simulink model "hardware5"  (R2021a)
settings: Solver=FixedStepAuto  StartTime=0.0  StopTime=1  FixedStep=0.001  RelTol=1e-3
undefined symbols (not defined in the file or in its folder): DiscIntNeverNeededParam
libraries: simulink x3
settings Model: Creator=acre  LastModifiedBy=acre
settings OptimizationCC: BlockReduction=off  OptimizeBlockIOStorage=off

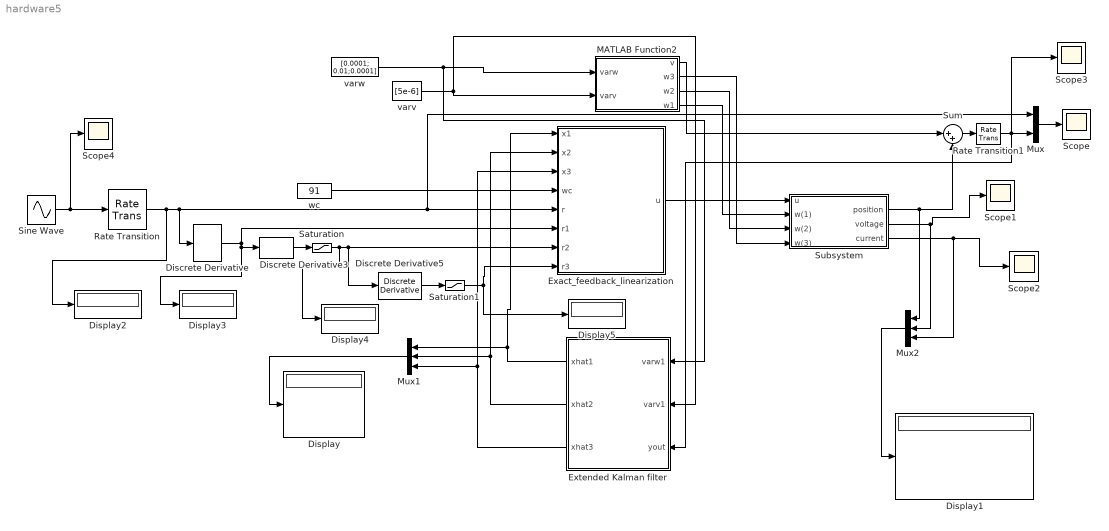
== system hardware5 ==
  Discrete Derivative : simulink/Discrete/Discrete Derivative  gainval=1.0  ICPrevScaledInput=0  OutMin=[]  OutMax=[]  OutDataType=fixdt(1, 16)  OutScaling=2^-10  DoSatur=off
  Discrete Derivative3 : simulink/Discrete/Discrete Derivative  gainval=1.0  ICPrevScaledInput=0  OutMin=[-1]  OutMax=[1]  OutDataType=fixdt(1, 16)  OutScaling=2^-10  DoSatur=on
      settings: LockScale=on
  Discrete Derivative5 : simulink/Discrete/Discrete Derivative  gainval=1.0  ICPrevScaledInput=0  OutMin=[]  OutMax=[]  OutDataType=fixdt(1, 16)  OutScaling=2^-10  DoSatur=off
  Display{,1..5} (6 alike) : Display
  Exact_feedback_linearization : Subsystem
  Extended Kalman filter : Subsystem
  MATLAB Function2 : MATLAB Function  TreatAsAtomicUnit=on
  Mux : Mux  Inputs=2
  Mux1 : Mux  Inputs=3
  Mux2 : Mux  Inputs=3
  Rate Transition : RateTransition
  Rate Transition1 : RateTransition
  Saturation : Saturate  UpperLimit=1  LowerLimit=-1
  Saturation1 : Saturate  UpperLimit=4  LowerLimit=-4
  Scope{,1..4} (5 alike) : Scope
  Sine Wave : Sin  Amplitude=0.1  Frequency=3  SampleTime=0
  Subsystem : Subsystem
  Sum : Sum  Inputs=|++
  varv : Constant  Value=[5e-6]  SampleTime=-1
  varw : Constant  Value=[0.0001; 0.01;0.0001]  SampleTime=-1
  wc : Constant  Value=91
  wires:
  Discrete Derivative3/1 -> Saturation/1
  Sine Wave/1 -> Scope4/1, Rate Transition/1
  Exact_feedback_linearization/1(u) -> Subsystem/1(u)
  Extended Kalman filter/3(xhat3) -> Mux1/3, Exact_feedback_linearization/3(x3)
  MATLAB Function2/2(w3) -> Subsystem/4(w(3))
  Mux1/1 -> Display/1
  Discrete Derivative5/1 -> Saturation1/1
  Rate Transition/1 -> Display2/1, Mux/1, Exact_feedback_linearization/5(r), Discrete Derivative/1
  Sum/1 -> Rate Transition1/1
  Mux/1 -> Scope/1
  Extended Kalman filter/1(xhat1) -> Exact_feedback_linearization/1(x1), Mux1/1
  MATLAB Function2/1(v) -> Sum/1
  varv/1 -> MATLAB Function2/2(varv), Extended Kalman filter/2(varv1)
  Saturation/1 -> Display4/1, Discrete Derivative5/1, Exact_feedback_linearization/7(r2)
  Rate Transition1/1 -> Extended Kalman filter/3(yout), Scope3/1, Mux/2
  Discrete Derivative/1 -> Display3/1, Discrete Derivative3/1, Exact_feedback_linearization/6(r1)
  wc/1 -> Exact_feedback_linearization/4(wc)
  MATLAB Function2/3(w2) -> Subsystem/3(w(2))
  Extended Kalman filter/2(xhat2) -> Mux1/2, Exact_feedback_linearization/2(x2)
  MATLAB Function2/4(w1) -> Subsystem/2(w(1))
  varw/1 -> Extended Kalman filter/1(varw1), MATLAB Function2/1(varw)
  Saturation1/1 -> Exact_feedback_linearization/8(r3), Display5/1
  Subsystem/1(position) -> Mux2/1, Sum/2
  Subsystem/2(voltage) -> Mux2/2, Scope1/1
  Subsystem/3(current) -> Mux2/3, Scope2/1
  Mux2/1 -> Display1/1

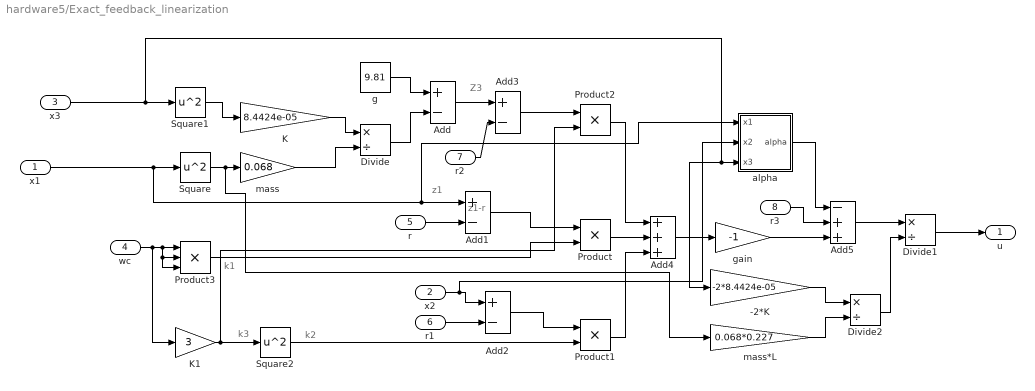
== system hardware5/Exact_feedback_linearization ==
  note: z1
  note: z1-r
  note: k3
  note: k2
  note: k1
  note: Z3
  x1 : Inport
  x2 : Inport  Port=2
  x3 : Inport  Port=3
  wc : Inport  Port=4
  r : Inport  Port=5
  r1 : Inport  Port=6
  r2 : Inport  Port=7
  r3 : Inport  Port=8
  -2*K : Gain  Gain=-2*8.4424e-05
  Add{,1..3} (4 alike) : Sum  Inputs=+-
  Add4 : Sum  Inputs=+++
  Add5 : Sum  Inputs=-++
  Divide : Product  Inputs=*/
  Divide1 : Product  Inputs=*/
  Divide2 : Product  Inputs=*/
  K : Gain  Gain=8.4424e-05
  K1 : Gain  Gain=3
  Product : Product
  Product1 : Product
  Product2 : Product
  Product3 : Product  Inputs=3
  Square : Math  Operator=square  SaturateOnIntegerOverflow=on
  Square1 : Math  Operator=square  SaturateOnIntegerOverflow=on
  Square2 : Math  Operator=square  SaturateOnIntegerOverflow=on
  alpha : Subsystem
  g : Constant  Value=9.81
  gain : Gain  Gain=-1
  mass : Gain  Gain=0.068
  mass*L : Gain  Gain=0.068*0.227
  u : Outport
  wires:
  g/1 -> Add/1
  Divide/1 -> Add/2
  Square1/1 -> K/1
  K/1 -> Divide/1
  mass/1 -> Divide/2
  wc/1 -> Product3/3, Product3/2, Product3/1, K1/1
  K1/1 -> Product2/2, Square2/1
  r/1 -> Add1/2
  Add1/1 -> Product/1
  Product3/1 -> Product/2
  r1/1 -> Add2/2
  x2/1 -> alpha/2(x2), Add2/1
  Add2/1 -> Product1/1
  Square2/1 -> Product1/2
  Add/1 -> Add3/1
  r2/1 -> Add3/2
  Add3/1 -> Product2/1
  Product2/1 -> Add4/1
  Product/1 -> Add4/2
  Product1/1 -> Add4/3
  Add4/1 -> gain/1
  gain/1 -> Add5/3
  r3/1 -> Add5/2
  Add5/1 -> Divide1/1
  Divide1/1 -> u/1
  Square/1 -> mass*L/1, mass/1
  -2*K/1 -> Divide2/1
  mass*L/1 -> Divide2/2
  Divide2/1 -> Divide1/2
  alpha/1(alpha) -> Add5/1
  x1/1 -> alpha/1(x1), Add1/1, Square/1
  x3/1 -> alpha/3(x3), -2*K/1, Square1/1

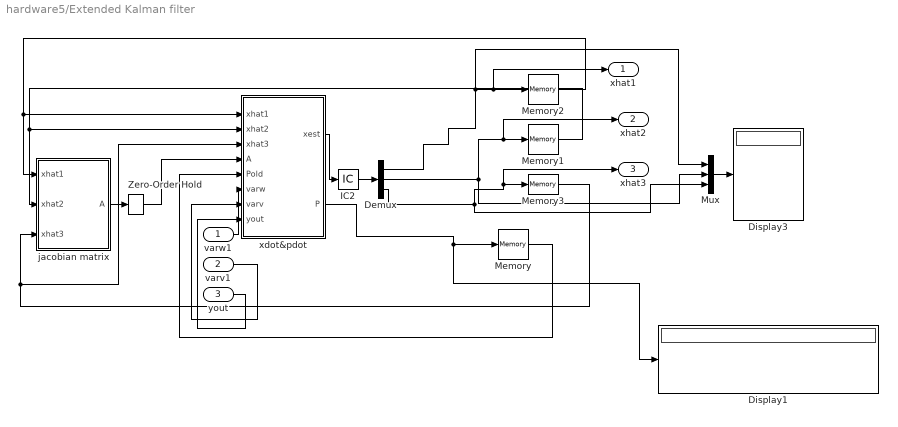
== system hardware5/Extended Kalman filter ==
  varw1 : Inport
  varv1 : Inport  Port=2
  yout : Inport  Port=3
  Demux : Demux  Outputs=3
  Display1 : Display
  Display3 : Display
  IC2 : InitialCondition  Value=[0.0095;0;0.84]
  Memory : Memory  InitialCondition=[0.00003 0 0;0 0.1 0;0 0 10]
  Memory1 : Memory  InitialCondition=0.0001
  Memory2 : Memory  InitialCondition=0.0095
  Memory3 : Memory  InitialCondition=0.84
  Mux : Mux  Inputs=3
  Zero-Order Hold : ZeroOrderHold  SampleTime=0.001
  jacobian matrix : MATLAB Function  TreatAsAtomicUnit=on
  xdot&pdot : MATLAB Function  TreatAsAtomicUnit=on
  xhat1 : Outport
  xhat2 : Outport  Port=2
  xhat3 : Outport  Port=3
  wires:
  varv1/1 -> xdot&pdot/7(varv)
  varw1/1 -> xdot&pdot/6(varw)
  Memory1/1 -> jacobian matrix/2(xhat2), xdot&pdot/2(xhat2)
  xdot&pdot/1(xest) -> IC2/1
  Memory2/1 -> jacobian matrix/1(xhat1), xdot&pdot/1(xhat1)
  Memory3/1 -> jacobian matrix/3(xhat3), xdot&pdot/3(xhat3)
  jacobian matrix/1(A) -> Zero-Order Hold/1
  Memory/1 -> xdot&pdot/5(Pold)
  yout/1 -> xdot&pdot/8(yout)
  Mux/1 -> Display3/1
  xdot&pdot/2(P) -> Display1/1, Memory/1
  Zero-Order Hold/1 -> xdot&pdot/4(A)
  Demux/1 -> Mux/1, xhat1/1, Memory2/1
  Demux/2 -> xhat2/1, Memory1/1, Mux/2
  Demux/3 -> Memory3/1, xhat3/1, Mux/3
  IC2/1 -> Demux/1

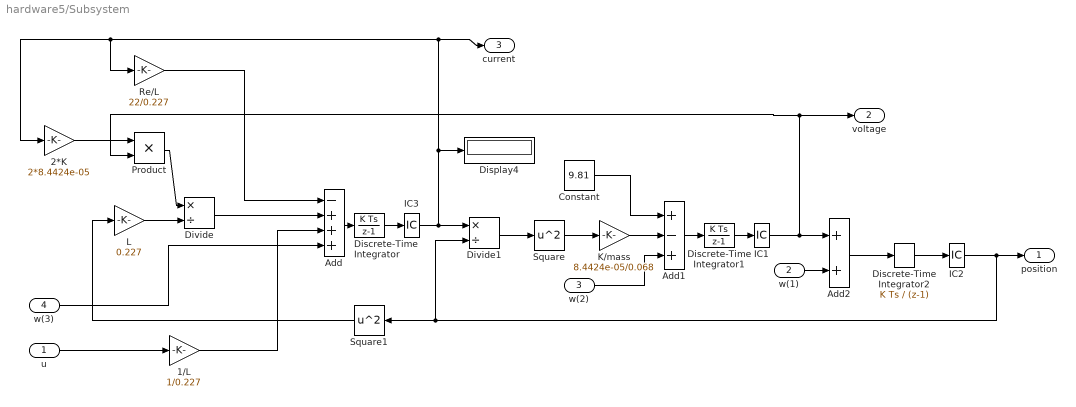
== system hardware5/Subsystem ==
  u : Inport
  w(1) : Inport  Port=2
  w(2) : Inport  Port=3
  w(3) : Inport  Port=4
  1/L : Gain  Gain=1/0.227
  2*K : Gain  Gain=2*8.4424e-05
  Add : Sum  Inputs=-+++
  Add1 : Sum  Inputs=+-+
  Add2 : Sum
  Constant : Constant  Value=9.81  SampleTime=-1
  Discrete-Time Integrator : DiscreteIntegrator  SampleTime=-1  UpperSaturationLimit=100  LowerSaturationLimit=-100  ICPrevOutput=DiscIntNeverNeededParam  ICPrevScaledInput=DiscIntNeverNeededParam
  Discrete-Time Integrator1 : DiscreteIntegrator  SampleTime=-1  UpperSaturationLimit=50  LowerSaturationLimit=-50  ICPrevOutput=DiscIntNeverNeededParam  ICPrevScaledInput=DiscIntNeverNeededParam
  Discrete-Time Integrator2 : DiscreteIntegrator  SampleTime=-1  UpperSaturationLimit=5  LowerSaturationLimit=-5  ICPrevOutput=DiscIntNeverNeededParam  ICPrevScaledInput=DiscIntNeverNeededParam
  Display4 : Display
  Divide : Product  Inputs=*/
  Divide1 : Product  Inputs=*/
  IC1 : InitialCondition  Value=0
  IC2 : InitialCondition  Value=0.009
  IC3 : InitialCondition  Value=0.8
  K/mass : Gain  Gain=8.4424e-05/0.068
  L : Gain  Gain=0.227
  Product : Product
  Re/L : Gain  Gain=22/0.227
  Square : Math  Operator=square  SaturateOnIntegerOverflow=on
  Square1 : Math  Operator=square  SaturateOnIntegerOverflow=on
  position : Outport
  voltage : Outport  Port=2
  current : Outport  Port=3
  wires:
  1/L/1 -> Add/3
  Add/1 -> Discrete-Time Integrator/1
  Re/L/1 -> Add/1
  2*K/1 -> Product/1
  w(3)/1 -> Add/4
  Divide/1 -> Add/2
  Product/1 -> Divide/1
  L/1 -> Divide/2
  Constant/1 -> Add1/1
  K/mass/1 -> Add1/2
  Square/1 -> K/mass/1
  Divide1/1 -> Square/1
  w(2)/1 -> Add1/3
  Add1/1 -> Discrete-Time Integrator1/1
  Discrete-Time Integrator1/1 -> IC1/1
  w(1)/1 -> Add2/2
  Add2/1 -> Discrete-Time Integrator2/1
  Discrete-Time Integrator2/1 -> IC2/1
  u/1 -> 1/L/1
  Square1/1 -> L/1
  Discrete-Time Integrator/1 -> IC3/1
  IC3/1 -> Divide1/1, Display4/1, current/1, Re/L/1, 2*K/1
  IC1/1 -> Product/2, voltage/1, Add2/1
  IC2/1 -> position/1, Divide1/2, Square1/1

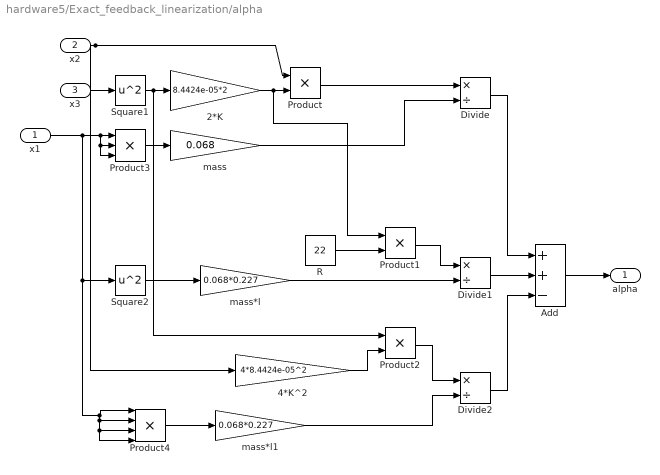
== system hardware5/Exact_feedback_linearization/alpha ==
  x1 : Inport
  x2 : Inport  Port=2
  x3 : Inport  Port=3
  2*K : Gain  Gain=8.4424e-05*2
  4*K^2 : Gain  Gain=4*8.4424e-05^2
  Add : Sum  Inputs=++-
  Divide : Product  Inputs=*/
  Divide1 : Product  Inputs=*/
  Divide2 : Product  Inputs=*/
  Product : Product
  Product1 : Product
  Product2 : Product
  Product3 : Product  Inputs=3
  Product4 : Product  Inputs=4
  R : Constant  Value=22
  Square1 : Math  Operator=square  SaturateOnIntegerOverflow=on
  Square2 : Math  Operator=square  SaturateOnIntegerOverflow=on
  mass : Gain  Gain=0.068
  mass*l : Gain  Gain=0.068*0.227
  mass*l1 : Gain  Gain=0.068*0.227
  alpha : Outport
  wires:
  Add/1 -> alpha/1
  x3/1 -> Square1/1
  x2/1 -> Product/1, 4*K^2/1
  Product/1 -> Divide/1
  mass/1 -> Divide/2
  Product3/1 -> mass/1
  x1/1 -> Product3/3, Product3/2, Product3/1, Product4/1, Product4/2, Product4/3, Product4/4, Square2/1
  Divide/1 -> Add/1
  Square1/1 -> Product2/1, 2*K/1
  2*K/1 -> Product1/1, Product/2
  Product1/1 -> Divide1/1
  R/1 -> Product1/2
  Square2/1 -> mass*l/1
  mass*l/1 -> Divide1/2
  Divide1/1 -> Add/2
  Product4/1 -> mass*l1/1
  mass*l1/1 -> Divide2/2
  Product2/1 -> Divide2/1
  4*K^2/1 -> Product2/2
  Divide2/1 -> Add/3

== matlab function hardware5/Extended Kalman filter/xdot&pdot ==
  data: xhat1 input; xest output; xhat2 input; xhat3 input; A input; Pold input; P output; varw input; varv input; yout input
function [xest, P] = fcn(xhat1,xhat2,xhat3,A,Pold,varw,varv,yout)
x0 = 0.009;                             %initial position in meter
mass = 0.068;                           %Kg (mass of the ball))
g = 9.81;
L0 = 0.018761;                           %Hertz
L=0.227;                                %Hertz
K = (x0*L0)/2;                           %electromagnet force constant
Re= 22;                                  %ohms
Lm  = eye(3);
Q = diag(varw);
H = [1 0 0];
M = [1 0 0];
R = diag(varv);
xhat = [xhat1;xhat2;xhat3];
P = A*Pold*A' +Lm*Q*Lm';
xest = A*xhat;
Kal = P*H'/(H*P*H'+M*R*M');
xest = xest +Kal*(yout-xest(1));
P = (eye(size(Kal,1))- Kal*H)*P;

== matlab function hardware5/Extended Kalman filter/jacobian matrix ==
  data: xhat1 input; A output; xhat2 input; xhat3 input
function A = fcn(xhat1,xhat2,xhat3)
dt = 0.001;
x0 = 0.009;                               %initial position in meter
mass = 0.068;                            %Kg (mass of the ball))
g = 9.81;
L0 = 0.018761;                          %Henry (Kg)(m^2)(s^-2)(A^-2)
%L0 = -3.1269375;                         %Henry (Kg)(m)(V)(s^-2)(A^-2)
Lind=0.227;                              %Henry(in terms of x as a meter)
%Lind=-37.83459;                              %Henry(in terms of x as voltage)
K = (x0*L0)/2;                          %electromagnet force constant
Re= 22;  
 A21 = ((2*K*(xhat3^2))/(mass*(xhat1^3)));
    A23 = (-2*K*xhat3)/(mass*(xhat1^2));
    A31 = (-4*K*xhat3*xhat2)/(Lind*xhat1^3);
    A32 = (2*K*xhat3)/(Lind*xhat1^2);
    A33 = (-Re/Lind)+((2*K*xhat2)/(Lind*xhat1^2));
    A = [0 1 0;A21 0 A23;A31 A32 A33];

== matlab function hardware5/MATLAB Function2 ==
  data: v output; varw input; varv input; w3 output; w2 output; w1 output
function [v,w3,w2,w1] = noise(varw,varv)
w1 = wgn(1,1,varw(1),'linear');
w2 =wgn(1,1,varw(2),'linear'); 
w3 = wgn(1,1,varw(3),'linear');
v = wgn(1,1,varv,'linear');
